simulink model "gm_Sementation_8K"  (R2019a)
settings: Solver=FixedStepDiscrete  StartTime=0.0  StopTime=Ts_240p*20  RelTol=1e-3
InitFcn:
  | Ts = 1e-3;
  | Ts_240p = 402*324*Ts;
  | Ts_480p = 525*800*Ts;
undefined symbols (not defined in the file or in its folder): gray, Rec, SDTV
libraries: hdlsllib x14, visionhdlio x2, visionhdlconversions x2, dspvision x1
settings Model: ModifiedByFormat=The MathWorks Inc.  Creator=The MathWorks, Inc.  LastModifiedBy=The MathWorks Inc.
settings DataIOCC: LimitDataPoints=on  SaveFormat=Array  SaveOutput=off  SaveTime=off  ReturnWorkspaceOutputs=off
settings OptimizationCC: BlockReduction=off  ConditionallyExecuteInputs=off  DefaultParameterBehavior=Inlined  LifeSpan=inf
settings DebuggingCC: AlgebraicLoopMsg=error  SolverPrmCheckMsg=warning  InheritedTsInSrcMsg=none  SingleTaskRateTransMsg=error  ParameterPrecisionLossMsg=none  AllowSymbolicDim=off  SFUnexpectedBacktrackingDiag=warning  SFNoUnconditionalDefaultTransitionDiag=warning  SFExecutionAtInitializationDiag=none  IntegerSaturationMsg=none  ArithmeticOperatorsInVariantConditions=warning
settings HardwareCC: ProdBitPerPointer=32  ProdBitPerSizeT=32  ProdBitPerPtrDiffT=32  ProdLargestAtomicFloat=None  ProdIntDivRoundTo=Undefined  ProdEndianess=Unspecified  ProdWordSize=32  ProdHWDeviceType=ASIC/FPGA->ASIC/FPGA  ProdEqTarget=off
settings ModelReferenceCC: PropagateSignalLabelsOutOfModel=off
settings SFSimCC: SimUseLocalCustomCode=off
settings RTWCC: RTWUseLocalCustomCode=off
settings CodeAppCC: StateflowObjectComments=on
settings GRTTargetCC: TargetLangStandard=C89/C90 (ANSI)  GeneratePreprocessorConditionals=Disable all
settings ConfigComp: CovMetricSettings=dw  CovHtmlReporting=on  CovSaveCumulativeToWorkspaceVar=on  CovSaveSingleToWorkspaceVar=on  CovShowResultsExplorer=off  CovExternalEMLEnable=off  CovSFcnEnable=off

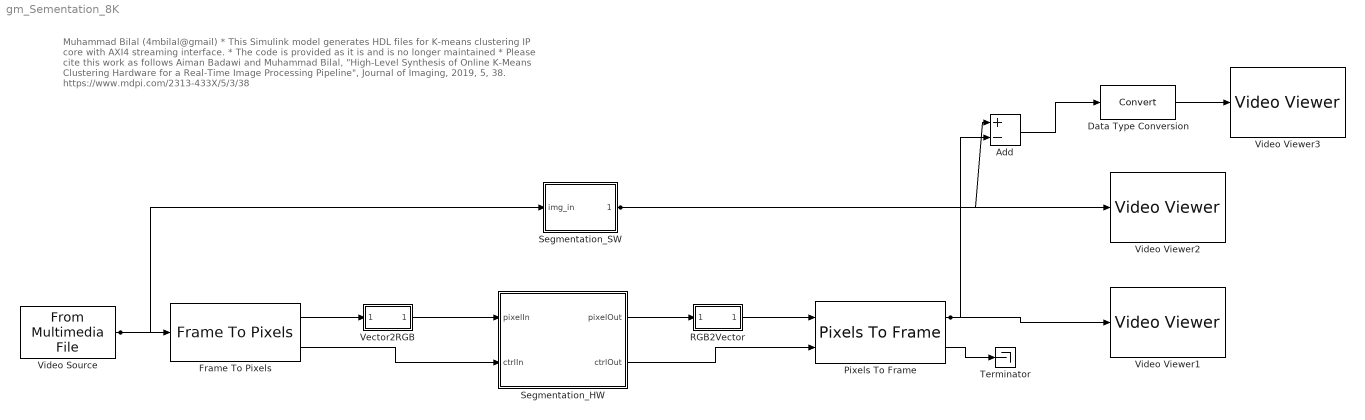
== system gm_Sementation_8K ==
  note: Muhammad Bilal (4mbilal@gmail)
      |
      | * This Simulink model generates HDL files for K-means clustering IP core with AXI4 streaming interface.
      |
      | * The code is provided as it is and is no longer maintained
      |
      | * Please cite this work as follows
      | Aiman Badawi and Muhammad Bilal, "High-Level Synthesis of Online K-Means Clustering Hardware for a Real-Time Image Processing Pipeline", Journal of Imaging, 2019, 5, 38.
      | https://www.mdpi.com/2313-433X/5/3/38
  Add : Sum  Inputs=+-
  Data Type Conversion : DataTypeConversion
  Frame To Pixels : visionhdlio/Frame To Pixels  NumComponents=3  VideoFormat=240p  ActivePixelsPerLine=32  ActiveVideoLines=18  TotalPixelsPerLine=42  TotalVideoLines=28  StartingActiveLine=6  FrontPorch=5  SampleTime=0
      settings: SourceProductName=Vision HDL Toolbox  SourceProductBaseCode=VT
  Pixels To Frame : visionhdlio/Pixels To Frame  NumComponents=3  VideoFormat=240p  ActivePixelsPerLine=32  ActiveVideoLines=18  TotalPixelsPerLine=42  TotalVideoLines=28
      settings: SourceProductName=Vision HDL Toolbox  SourceProductBaseCode=VT
  RGB2Vector : Subsystem
  Segmentation_HW : Subsystem  TreatAsAtomicUnit=on
  Segmentation_SW : MATLAB Function  TreatAsAtomicUnit=on
  Terminator : Terminator
  Vector2RGB : Subsystem
  Video Source : dspvision/From Multimedia File  inputFilename=E:\RnD\Current_Projects\Musawwir\Frameworks\HW\Musawwir_HW_Zedboard\Custom_IP_Cores\Matlab\Segmentation\images\mountain.jpg  readRange=[1 Inf]  loop=on  numPlays=inf  outputStreams=Video only  videoDataType=uint8  audioDataType=int16  inheritSampleTime=off  userDefinedSampleTime=Ts_240p  noAudioOutput=off  isIntensityVideo=off  fourcc=RGB  colorVideoFormat=One multidimensional signal  outputEOF=off  dataOrg=Column-major  audioFrameSize=1024  computeAudioFrameSize=off  outSamplingMode=Sample based
      settings: SourceProductName=Computer Vision Toolbox  SourceProductBaseCode=VP
  Video Viewer1 : VideoViewer  colormapValue=gray(256)  FigPos=[54.6 658.8 498.4 402.4]
  Video Viewer2 : VideoViewer  colormapValue=gray(256)  FigPos=[554.6 659.6 498.4 402.4]
  Video Viewer3 : VideoViewer  colormapValue=gray(256)  FigPos=[1020.2 514 498.4 402.4]
  wires:
  Data Type Conversion/1 -> Video Viewer3/1
  Add/1 -> Data Type Conversion/1
  Segmentation_SW/1(img_out) -> Video Viewer2/1, Add/1
  Segmentation_HW/2(ctrlOut) -> Pixels To Frame/2
  RGB2Vector/1(RGBVector) -> Pixels To Frame/1
  Frame To Pixels/1 -> Vector2RGB/1(RGBVector)
  Frame To Pixels/2 -> Segmentation_HW/2(ctrlIn)
  Video Source/1 -> Frame To Pixels/1, Segmentation_SW/1(img_in)
  Segmentation_HW/1(pixelOut) -> RGB2Vector/1(RGB)
  Vector2RGB/1(RGB) -> Segmentation_HW/1(pixelIn)
  Pixels To Frame/1 -> Video Viewer1/1, Add/2
  Pixels To Frame/2 -> Terminator/1

== system gm_Sementation_8K/RGB2Vector ==
  note: RGB represented in
      | 32'hFFRRGGBB
  RGB : Inport
  Bit Slice : hdlsllib/Logic and Bit Operations/Bit Slice  lidx=23  ridx=16
  Bit Slice1 : hdlsllib/Logic and Bit Operations/Bit Slice  lidx=15  ridx=8
  Bit Slice2 : hdlsllib/Logic and Bit Operations/Bit Slice  lidx=7  ridx=0
  Mux : Mux  Inputs=3
  Signal Specification : SignalSpecification
  Transpose : Math  Operator=transpose  SaturateOnIntegerOverflow=on
  RGBVector : Outport
  wires:
  Signal Specification/1 -> RGBVector/1
  Transpose/1 -> Signal Specification/1
  RGB/1 -> Bit Slice/1, Bit Slice1/1, Bit Slice2/1
  Bit Slice1/1 -> Mux/2
  Bit Slice2/1 -> Mux/3
  Bit Slice/1 -> Mux/1
  Mux/1 -> Transpose/1

== system gm_Sementation_8K/Segmentation_HW ==
  pixelIn : Inport  OutDataTypeStr=uint32  PortDimensions=1  SampleTime=0.001
  ctrlIn : Inport  Port=2  SampleTime=0.001
  Bit Concat : hdlsllib/Logic and Bit Operations/Bit Concat  numInputs=4
      settings: SourceProductName=HDL Coder  SourceProductBaseCode=HD
  Demux : Demux  Outputs=3
  FF : Constant  Value=255  OutDataTypeStr=uint8  SampleTime=Ts
  K-Means : Subsystem
  RGB2Vector : Subsystem
  pixelOut : Outport
  ctrlOut : Outport  Port=2
  wires:
  pixelIn/1 -> RGB2Vector/1(RGB)
  ctrlIn/1 -> K-Means/2(ctrlIn)
  Bit Concat/1 -> pixelOut/1
  Demux/1 -> Bit Concat/2
  Demux/2 -> Bit Concat/3
  Demux/3 -> Bit Concat/4
  FF/1 -> Bit Concat/1
  K-Means/1(pixelOut) -> Demux/1
  K-Means/2(ctrlOut) -> ctrlOut/1
  RGB2Vector/1(RGBVector) -> K-Means/1(pixelIn)

== system gm_Sementation_8K/Vector2RGB ==
  note: Encode RGB into 32 bit representation
      | 32'hFFRRGGBB
  RGBVector : Inport
  Bit Concat : hdlsllib/Logic and Bit Operations/Bit Concat  numInputs=4
      settings: SourceProductName=HDL Coder  SourceProductBaseCode=HD
  Demux : Demux  Outputs=3
  FF : Constant  Value=255  OutDataTypeStr=uint8  SampleTime=Ts
  RGB : Outport
  wires:
  Demux/3 -> Bit Concat/4
  Demux/2 -> Bit Concat/3
  Demux/1 -> Bit Concat/2
  FF/1 -> Bit Concat/1
  RGBVector/1 -> Demux/1
  Bit Concat/1 -> RGB/1

== system gm_Sementation_8K/Segmentation_HW/K-Means ==
  pixelIn : Inport  OutDataTypeStr=uint8  PortDimensions=[3]  SampleTime=0.001
  ctrlIn : Inport  Port=2  SampleTime=0.001
  Clustering : Subsystem
  Color Space Converter : visionhdlconversions/Color Space Converter  Conversion=RGB to YCbCr  ConversionStandard=Rec. 601 (SDTV)  ScanningStandard=1250/50/2:1  SimulateUsing=Code generation
      settings: SourceProductName=Vision HDL Toolbox  SourceProductBaseCode=VT
  Color Space Converter1 : visionhdlconversions/Color Space Converter  Conversion=YCbCr to RGB  ConversionStandard=Rec. 601 (SDTV)  ScanningStandard=1250/50/2:1  SimulateUsing=Code generation
      settings: SourceProductName=Vision HDL Toolbox  SourceProductBaseCode=VT
  Comparisons : Subsystem
  Data Type Conversion1 : DataTypeConversion  OutDataTypeStr=uint8  RndMeth=Nearest  SampleTime=0.001
  Data Type Conversion2 : DataTypeConversion  OutDataTypeStr=fixdt(1, 18, 8)  RndMeth=Nearest  SampleTime=0.001
  pixelOut : Outport
  ctrlOut : Outport  Port=2
  wires:
  pixelIn/1 -> Color Space Converter/1
  ctrlIn/1 -> Color Space Converter/2
  Clustering/1(K_out) -> Comparisons/2(Ks)
  Color Space Converter/1 -> Data Type Conversion2/1
  Color Space Converter/2 -> Clustering/3(Ctrl), Color Space Converter1/2
  Color Space Converter1/1 -> pixelOut/1
  Color Space Converter1/2 -> ctrlOut/1
  Comparisons/1(K_out) -> Data Type Conversion1/1
  Comparisons/2(Address) -> Clustering/1(K_addr)
  Data Type Conversion1/1 -> Color Space Converter1/1
  Data Type Conversion2/1 -> Clustering/2(RGB_pixel), Comparisons/1(RGB_pixel)

== system gm_Sementation_8K/Segmentation_HW/RGB2Vector ==
  RGB : Inport  OutDataTypeStr=uint32  PortDimensions=1  SampleTime=0.001
  Bit Slice : hdlsllib/Logic and Bit Operations/Bit Slice  lidx=23  ridx=16
  Bit Slice1 : hdlsllib/Logic and Bit Operations/Bit Slice  lidx=15  ridx=8
  Bit Slice2 : hdlsllib/Logic and Bit Operations/Bit Slice  lidx=7  ridx=0
  Mux : Mux  Inputs=3
  RGBVector : Outport
  wires:
  RGB/1 -> Bit Slice2/1, Bit Slice1/1, Bit Slice/1
  Bit Slice/1 -> Mux/1
  Bit Slice1/1 -> Mux/2
  Bit Slice2/1 -> Mux/3
  Mux/1 -> RGBVector/1

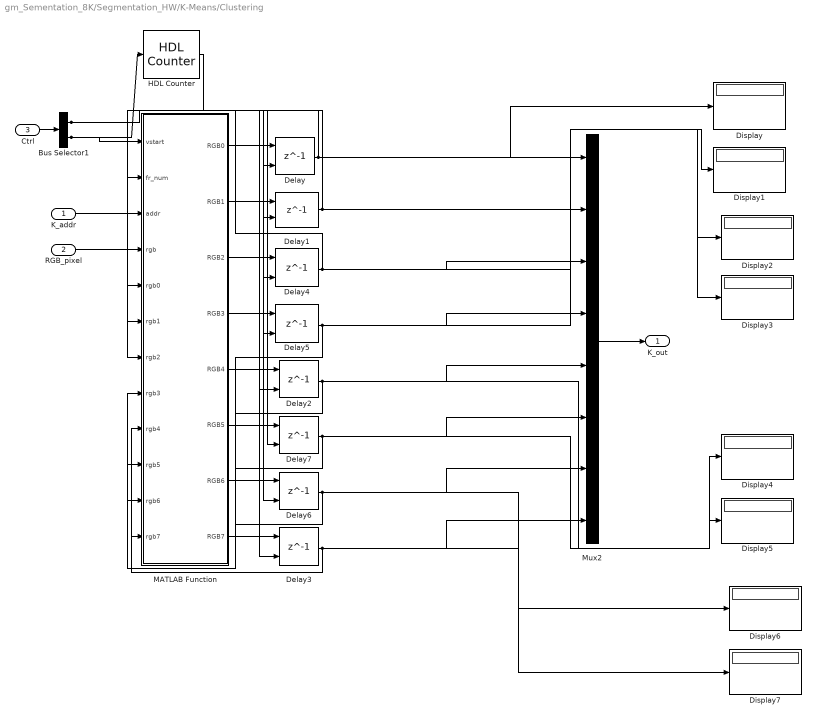
== system gm_Sementation_8K/Segmentation_HW/K-Means/Clustering ==
  K_addr : Inport  OutDataTypeStr=fixdt(0, 3, 0)  PortDimensions=1  SampleTime=0.001
  RGB_pixel : Inport  Port=2  OutDataTypeStr=fixdt(1, 18, 8)  PortDimensions=[1 3]  SampleTime=0.001
  Ctrl : Inport  Port=3  SampleTime=0.001
  Bus Selector1 : BusSelector  OutputSignals=valid,vStart
  Delay{,1..7} (8 alike) : Delay  DelayLength=1  InitialCondition=0  ShowEnablePort=on
      settings: InputPortMap=u0,e6
  Display{,1..7} (8 alike) : Display
  HDL Counter : hdlsllib/Sources/HDL Counter  CountType=Free running  CountInit=0  CountStep=1  CountMax=4  CountFromType=Initial value  CountFrom=0  CountResetPort=off  CountLoadPort=off  CountEnbPort=on  CountDirPort=off  CountDataType=Unsigned  CountWordLen=12  CountFracLen=0  CountSampTime=1
      settings: SourceProductBaseCode=HD
  MATLAB Function : Subsystem
  Mux2 : Mux  Inputs=8
  K_out : Outport
  wires:
  K_addr/1 -> MATLAB Function/3(addr)
  RGB_pixel/1 -> MATLAB Function/4(rgb)
  Ctrl/1 -> Bus Selector1/1
  Bus Selector1/1 -> Delay7/2, Delay6/2, Delay5/2, Delay4/2, Delay3/2, Delay2/2, Delay1/2, Delay/2
  Bus Selector1/2 -> HDL Counter/1, MATLAB Function/1(vstart)
  Delay/1 -> Mux2/1, Display/1, MATLAB Function/5(rgb0)
  Delay1/1 -> Mux2/2, Display1/1, MATLAB Function/6(rgb1)
  Delay2/1 -> Mux2/5, Display4/1, MATLAB Function/9(rgb4)
  Delay3/1 -> Mux2/8, Display7/1, MATLAB Function/12(rgb7)
  Delay4/1 -> Mux2/3, Display2/1, MATLAB Function/7(rgb2)
  Delay5/1 -> Mux2/4, Display3/1, MATLAB Function/8(rgb3)
  Delay6/1 -> Mux2/7, Display6/1, MATLAB Function/11(rgb6)
  Delay7/1 -> Mux2/6, Display5/1, MATLAB Function/10(rgb5)
  HDL Counter/1 -> MATLAB Function/2(fr_num)
  MATLAB Function/1(RGB0) -> Delay/1
  MATLAB Function/2(RGB1) -> Delay1/1
  MATLAB Function/3(RGB2) -> Delay4/1
  MATLAB Function/4(RGB3) -> Delay5/1
  MATLAB Function/5(RGB4) -> Delay2/1
  MATLAB Function/6(RGB5) -> Delay7/1
  MATLAB Function/7(RGB6) -> Delay6/1
  MATLAB Function/8(RGB7) -> Delay3/1
  Mux2/1 -> K_out/1

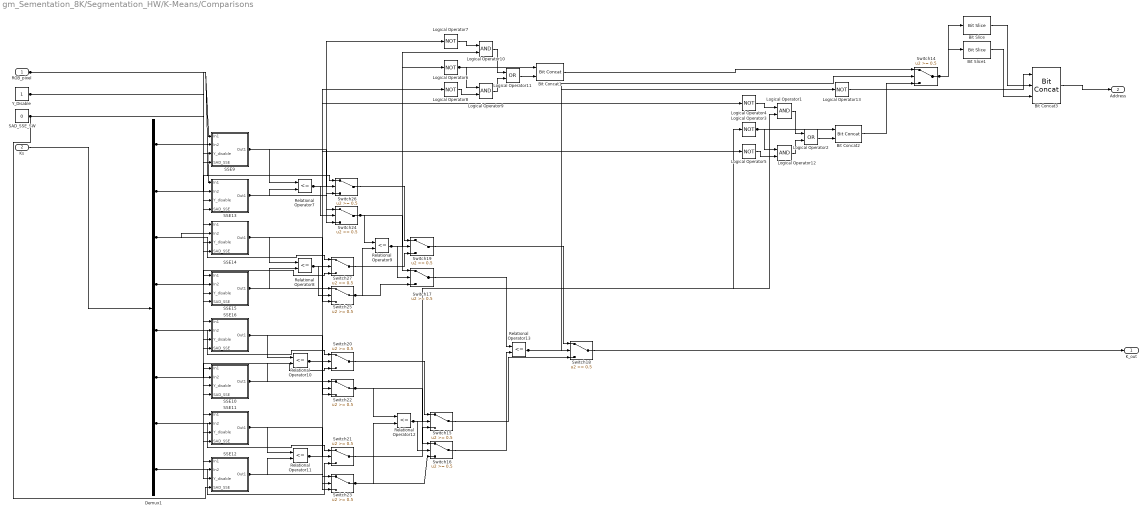
== system gm_Sementation_8K/Segmentation_HW/K-Means/Comparisons ==
  RGB_pixel : Inport  OutDataTypeStr=fixdt(1, 18, 8)  PortDimensions=[1 3]  SampleTime=0.001
  Ks : Inport  Port=2  OutDataTypeStr=fixdt(1, 18, 8)  PortDimensions=[1 24]  SampleTime=0.001
  Bit Concat1 : hdlsllib/Logic and Bit Operations/Bit Concat  numInputs=2
      settings: SourceProductName=HDL Coder  SourceProductBaseCode=HD
  Bit Concat2 : hdlsllib/Logic and Bit Operations/Bit Concat  numInputs=2
      settings: SourceProductName=HDL Coder  SourceProductBaseCode=HD
  Bit Concat3 : hdlsllib/Logic and Bit Operations/Bit Concat  numInputs=3
      settings: SourceProductName=HDL Coder  SourceProductBaseCode=HD
  Bit Slice : hdlsllib/Logic and Bit Operations/Bit Slice  lidx=1  ridx=1
  Bit Slice1 : hdlsllib/Logic and Bit Operations/Bit Slice  lidx=0  ridx=0
  Demux1 : Demux  Outputs=8
  Logical Operator{1,9..10,12} (4 alike) : Logic  AllPortsSameDT=off  OutDataTypeStr=boolean
  Logical Operator11 : Logic  Operator=OR  AllPortsSameDT=off  OutDataTypeStr=boolean
  Logical Operator{3..8,13} (7 alike) : Logic  Operator=NOT  AllPortsSameDT=off  OutDataTypeStr=boolean
  Logical Operator2 : Logic  Operator=OR  AllPortsSameDT=off  OutDataTypeStr=boolean
  Relational Operator{7..13} (7 alike) : RelationalOperator  Operator=<=  OutDataTypeStr=boolean  RndMeth=Nearest
  SAD_SSE_SW : Constant  Value=0  OutDataTypeStr=fixdt(1,18,8)
  SSE10 : Subsystem
  SSE11 : Subsystem
  SSE12 : Subsystem
  SSE13 : Subsystem
  SSE14 : Subsystem
  SSE15 : Subsystem
  SSE16 : Subsystem
  SSE9 : Subsystem
  Switch{14..27} (14 alike) : Switch  Threshold=0.5
  Y_Disable : Constant  OutDataTypeStr=fixdt(1,18,8)
  K_out : Outport
  Address : Outport  Port=2
  wires:
  RGB_pixel/1 -> SSE13/1(In1), SSE14/1(In1), SSE11/1(In1), SSE12/1(In1), SSE10/1(In1), SSE16/1(In1), SSE15/1(In1), SSE9/1(In1)
  Ks/1 -> Demux1/1
  Bit Concat1/1 -> Switch14/1
  Bit Concat2/1 -> Switch14/3
  Bit Concat3/1 -> Address/1
  Bit Slice/1 -> Bit Concat3/2
  Bit Slice1/1 -> Bit Concat3/3
  Demux1/1 -> Switch26/1, SSE9/2(In2)
  Demux1/2 -> Switch26/3, SSE13/2(In2)
  Demux1/3 -> Switch27/1, SSE14/2(In2)
  Demux1/4 -> Switch27/3, SSE15/2(In2)
  Demux1/5 -> Switch20/1, SSE16/2(In2)
  Demux1/6 -> Switch20/3, SSE10/2(In2)
  Demux1/7 -> Switch21/1, SSE11/2(In2)
  Demux1/8 -> Switch21/3, SSE12/2(In2)
  Logical Operator1/1 -> Logical Operator2/1
  Logical Operator10/1 -> Logical Operator11/1
  Logical Operator11/1 -> Bit Concat1/2
  Logical Operator12/1 -> Logical Operator2/2
  Logical Operator13/1 -> Bit Concat3/1
  Logical Operator2/1 -> Bit Concat2/2
  Logical Operator3/1 -> Logical Operator12/1, Bit Concat2/1
  Logical Operator4/1 -> Logical Operator1/1
  Logical Operator5/1 -> Logical Operator12/2
  Logical Operator6/1 -> Logical Operator9/1, Bit Concat1/1
  Logical Operator7/1 -> Logical Operator10/1
  Logical Operator8/1 -> Logical Operator9/2
  Logical Operator9/1 -> Logical Operator11/2
  Relational Operator10/1 -> Switch22/2, Switch20/2, Logical Operator4/1
  Relational Operator11/1 -> Switch23/2, Switch21/2, Logical Operator5/1
  Relational Operator12/1 -> Switch16/2, Switch15/2, Logical Operator3/1, Logical Operator1/2
  Relational Operator13/1 -> Switch18/2, Switch14/2, Logical Operator13/1
  Relational Operator7/1 -> Switch26/2, Switch24/2, Logical Operator7/1
  Relational Operator8/1 -> Switch27/2, Switch25/2, Logical Operator8/1
  Relational Operator9/1 -> Switch19/2, Switch17/2, Logical Operator6/1, Logical Operator10/2
  SAD_SSE_SW/1 -> SSE12/4(SAD_SSE), SSE11/4(SAD_SSE), SSE10/4(SAD_SSE), SSE16/4(SAD_SSE), SSE15/4(SAD_SSE), SSE14/4(SAD_SSE), SSE13/4(SAD_SSE), SSE9/4(SAD_SSE)
  SSE10/1(Out1) -> Switch22/3, Relational Operator10/2
  SSE11/1(Out1) -> Switch23/1, Relational Operator11/1
  SSE12/1(Out1) -> Switch23/3, Relational Operator11/2
  SSE13/1(Out1) -> Switch24/3, Relational Operator7/2
  SSE14/1(Out1) -> Switch25/1, Relational Operator8/1
  SSE15/1(Out1) -> Switch25/3, Relational Operator8/2
  SSE16/1(Out1) -> Switch22/1, Relational Operator10/1
  SSE9/1(Out1) -> Switch24/1, Relational Operator7/1
  Switch14/1 -> Bit Slice1/1, Bit Slice/1
  Switch15/1 -> Switch18/3
  Switch16/1 -> Relational Operator13/2
  Switch17/1 -> Relational Operator13/1
  Switch18/1 -> K_out/1
  Switch19/1 -> Switch18/1
  Switch20/1 -> Switch15/1
  Switch21/1 -> Switch15/3
  Switch22/1 -> Switch16/1, Relational Operator12/1
  Switch23/1 -> Switch16/3, Relational Operator12/2
  Switch24/1 -> Switch17/1, Relational Operator9/1
  Switch25/1 -> Switch17/3, Relational Operator9/2
  Switch26/1 -> Switch19/1
  Switch27/1 -> Switch19/3
  Y_Disable/1 -> SSE9/3(Y_disable), SSE13/3(Y_disable), SSE16/3(Y_disable), SSE11/3(Y_disable), SSE12/3(Y_disable), SSE10/3(Y_disable), SSE15/3(Y_disable), SSE14/3(Y_disable)

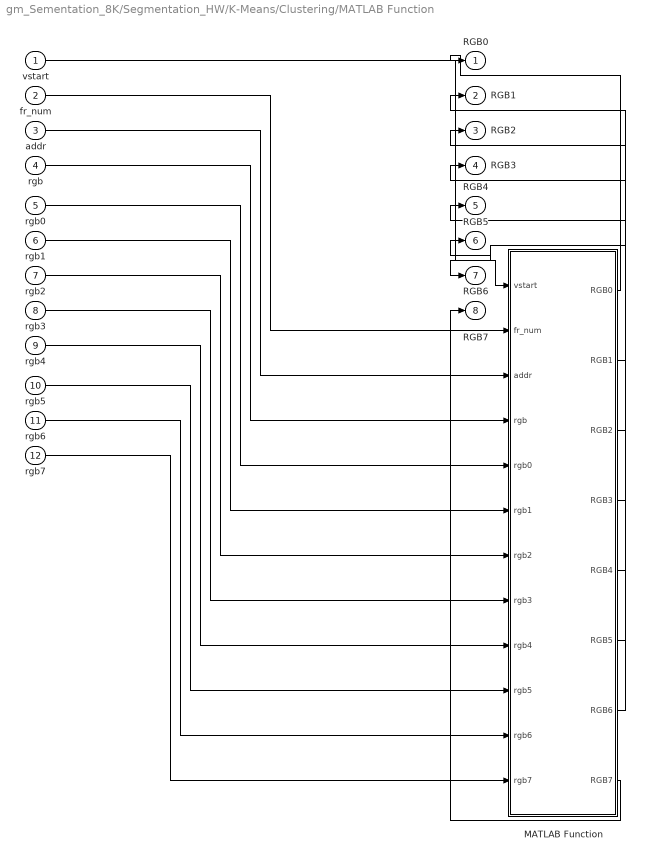
== system gm_Sementation_8K/Segmentation_HW/K-Means/Clustering/MATLAB Function ==
  vstart : Inport  OutDataTypeStr=boolean  PortDimensions=1  SampleTime=0.001
  fr_num : Inport  Port=2  OutDataTypeStr=fixdt(0, 12, 0)  PortDimensions=1  SampleTime=0.001
  addr : Inport  Port=3  OutDataTypeStr=fixdt(0, 3, 0)  PortDimensions=1  SampleTime=0.001
  rgb : Inport  Port=4  OutDataTypeStr=fixdt(1, 18, 8)  PortDimensions=[1 3]  SampleTime=0.001
  rgb0 : Inport  Port=5  OutDataTypeStr=fixdt(1, 18, 8)  PortDimensions=[1 3]  SampleTime=0.001
  rgb1 : Inport  Port=6  OutDataTypeStr=fixdt(1, 18, 8)  PortDimensions=[1 3]  SampleTime=0.001
  rgb2 : Inport  Port=7  OutDataTypeStr=fixdt(1, 18, 8)  PortDimensions=[1 3]  SampleTime=0.001
  rgb3 : Inport  Port=8  OutDataTypeStr=fixdt(1, 18, 8)  PortDimensions=[1 3]  SampleTime=0.001
  rgb4 : Inport  Port=9  OutDataTypeStr=fixdt(1, 18, 8)  PortDimensions=[1 3]  SampleTime=0.001
  rgb5 : Inport  Port=10  OutDataTypeStr=fixdt(1, 18, 8)  PortDimensions=[1 3]  SampleTime=0.001
  rgb6 : Inport  Port=11  OutDataTypeStr=fixdt(1, 18, 8)  PortDimensions=[1 3]  SampleTime=0.001
  rgb7 : Inport  Port=12  OutDataTypeStr=fixdt(1, 18, 8)  PortDimensions=[1 3]  SampleTime=0.001
  MATLAB Function : MATLAB Function  TreatAsAtomicUnit=on
  RGB0 : Outport
  RGB1 : Outport  Port=2
  RGB2 : Outport  Port=3
  RGB3 : Outport  Port=4
  RGB4 : Outport  Port=5
  RGB5 : Outport  Port=6
  RGB6 : Outport  Port=7
  RGB7 : Outport  Port=8
  wires:
  vstart/1 -> MATLAB Function/1(vstart)
  fr_num/1 -> MATLAB Function/2(fr_num)
  addr/1 -> MATLAB Function/3(addr)
  rgb/1 -> MATLAB Function/4(rgb)
  rgb0/1 -> MATLAB Function/5(rgb0)
  rgb1/1 -> MATLAB Function/6(rgb1)
  rgb2/1 -> MATLAB Function/7(rgb2)
  rgb3/1 -> MATLAB Function/8(rgb3)
  rgb4/1 -> MATLAB Function/9(rgb4)
  rgb5/1 -> MATLAB Function/10(rgb5)
  rgb6/1 -> MATLAB Function/11(rgb6)
  rgb7/1 -> MATLAB Function/12(rgb7)
  MATLAB Function/1(RGB0) -> RGB0/1
  MATLAB Function/2(RGB1) -> RGB1/1
  MATLAB Function/3(RGB2) -> RGB2/1
  MATLAB Function/4(RGB3) -> RGB3/1
  MATLAB Function/5(RGB4) -> RGB4/1
  MATLAB Function/6(RGB5) -> RGB5/1
  MATLAB Function/7(RGB6) -> RGB6/1
  MATLAB Function/8(RGB7) -> RGB7/1

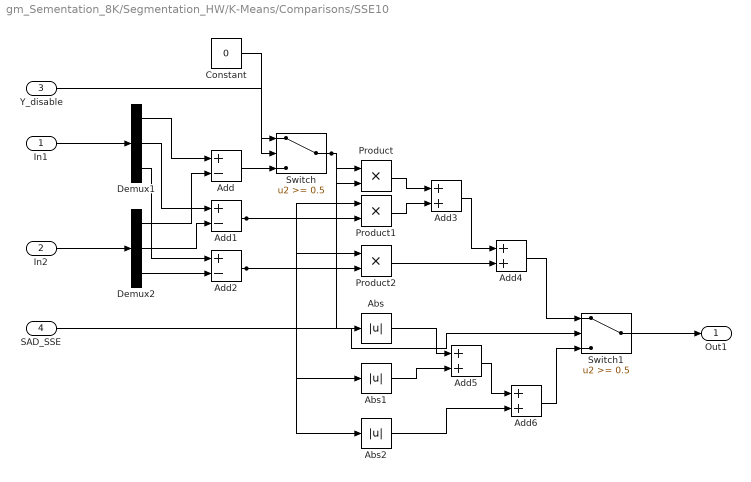
== system gm_Sementation_8K/Segmentation_HW/K-Means/Comparisons/SSE10 ==
  In1 : Inport  OutDataTypeStr=fixdt(1, 18, 8)  PortDimensions=[1 3]  SampleTime=0.001
  In2 : Inport  Port=2  OutDataTypeStr=fixdt(1, 18, 8)  PortDimensions=[1 3]  SampleTime=0.001
  Y_disable : Inport  Port=3  OutDataTypeStr=fixdt(1, 18, 8)  PortDimensions=1
  SAD_SSE : Inport  Port=4  OutDataTypeStr=fixdt(1, 18, 8)  PortDimensions=1
  Abs : Abs
  Abs1 : Abs
  Abs2 : Abs
  Add : Sum  Inputs=+-  OutDataTypeStr=Inherit: Inherit via back propagation
  Add1 : Sum  Inputs=+-  OutDataTypeStr=Inherit: Inherit via back propagation
  Add2 : Sum  Inputs=+-  OutDataTypeStr=Inherit: Inherit via back propagation
  Add{3..6} (4 alike) : Sum
  Constant : Constant  Value=0  OutDataTypeStr=fixdt(1,18,8)
  Demux1 : Demux  Outputs=3
  Demux2 : Demux  Outputs=3
  Product : Product
  Product1 : Product
  Product2 : Product
  Switch : Switch  Threshold=0.5
  Switch1 : Switch  Threshold=0.5
  Out1 : Outport
  wires:
  In1/1 -> Demux1/1
  In2/1 -> Demux2/1
  Y_disable/1 -> Switch/2
  SAD_SSE/1 -> Switch1/2
  Abs/1 -> Add5/1
  Abs1/1 -> Add5/2
  Abs2/1 -> Add6/2
  Add/1 -> Switch/3
  Add1/1 -> Product1/2, Product1/1, Abs1/1
  Add2/1 -> Product2/2, Product2/1, Abs2/1
  Add3/1 -> Add4/1
  Add4/1 -> Switch1/1
  Add5/1 -> Add6/1
  Add6/1 -> Switch1/3
  Constant/1 -> Switch/1
  Demux1/1 -> Add/1
  Demux1/2 -> Add1/1
  Demux1/3 -> Add2/1
  Demux2/1 -> Add/2
  Demux2/2 -> Add1/2
  Demux2/3 -> Add2/2
  Product/1 -> Add3/1
  Product1/1 -> Add3/2
  Product2/1 -> Add4/2
  Switch/1 -> Product/2, Product/1, Abs/1
  Switch1/1 -> Out1/1

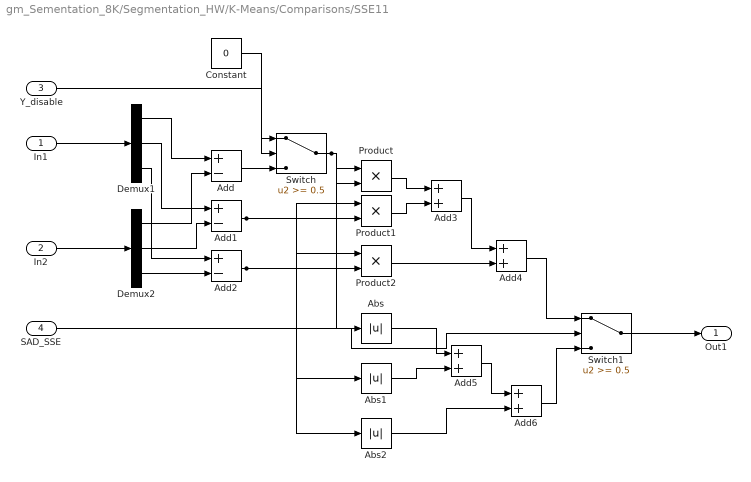
== system gm_Sementation_8K/Segmentation_HW/K-Means/Comparisons/SSE11 ==
  In1 : Inport  OutDataTypeStr=fixdt(1, 18, 8)  PortDimensions=[1 3]  SampleTime=0.001
  In2 : Inport  Port=2  OutDataTypeStr=fixdt(1, 18, 8)  PortDimensions=[1 3]  SampleTime=0.001
  Y_disable : Inport  Port=3  OutDataTypeStr=fixdt(1, 18, 8)  PortDimensions=1
  SAD_SSE : Inport  Port=4  OutDataTypeStr=fixdt(1, 18, 8)  PortDimensions=1
  Abs : Abs
  Abs1 : Abs
  Abs2 : Abs
  Add : Sum  Inputs=+-  OutDataTypeStr=Inherit: Inherit via back propagation
  Add1 : Sum  Inputs=+-  OutDataTypeStr=Inherit: Inherit via back propagation
  Add2 : Sum  Inputs=+-  OutDataTypeStr=Inherit: Inherit via back propagation
  Add{3..6} (4 alike) : Sum
  Constant : Constant  Value=0  OutDataTypeStr=fixdt(1,18,8)
  Demux1 : Demux  Outputs=3
  Demux2 : Demux  Outputs=3
  Product : Product
  Product1 : Product
  Product2 : Product
  Switch : Switch  Threshold=0.5
  Switch1 : Switch  Threshold=0.5
  Out1 : Outport
  wires:
  In1/1 -> Demux1/1
  In2/1 -> Demux2/1
  Y_disable/1 -> Switch/2
  SAD_SSE/1 -> Switch1/2
  Abs/1 -> Add5/1
  Abs1/1 -> Add5/2
  Abs2/1 -> Add6/2
  Add/1 -> Switch/3
  Add1/1 -> Product1/2, Product1/1, Abs1/1
  Add2/1 -> Product2/2, Product2/1, Abs2/1
  Add3/1 -> Add4/1
  Add4/1 -> Switch1/1
  Add5/1 -> Add6/1
  Add6/1 -> Switch1/3
  Constant/1 -> Switch/1
  Demux1/1 -> Add/1
  Demux1/2 -> Add1/1
  Demux1/3 -> Add2/1
  Demux2/1 -> Add/2
  Demux2/2 -> Add1/2
  Demux2/3 -> Add2/2
  Product/1 -> Add3/1
  Product1/1 -> Add3/2
  Product2/1 -> Add4/2
  Switch/1 -> Product/2, Product/1, Abs/1
  Switch1/1 -> Out1/1

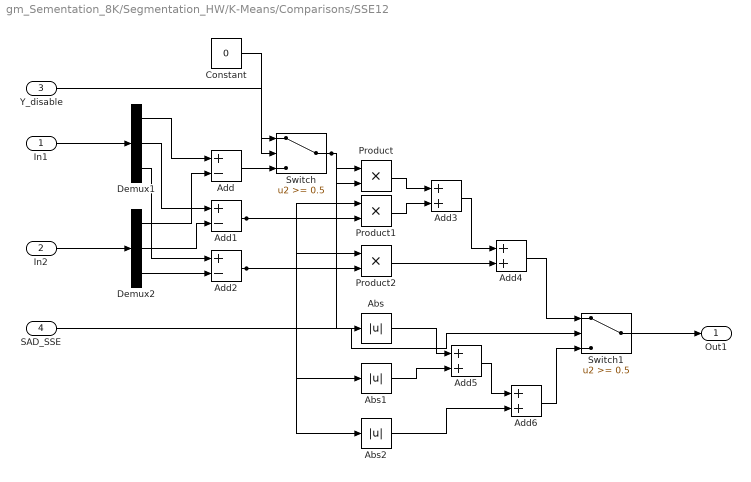
== system gm_Sementation_8K/Segmentation_HW/K-Means/Comparisons/SSE12 ==
  In1 : Inport  OutDataTypeStr=fixdt(1, 18, 8)  PortDimensions=[1 3]  SampleTime=0.001
  In2 : Inport  Port=2  OutDataTypeStr=fixdt(1, 18, 8)  PortDimensions=[1 3]  SampleTime=0.001
  Y_disable : Inport  Port=3  OutDataTypeStr=fixdt(1, 18, 8)  PortDimensions=1
  SAD_SSE : Inport  Port=4  OutDataTypeStr=fixdt(1, 18, 8)  PortDimensions=1
  Abs : Abs
  Abs1 : Abs
  Abs2 : Abs
  Add : Sum  Inputs=+-  OutDataTypeStr=Inherit: Inherit via back propagation
  Add1 : Sum  Inputs=+-  OutDataTypeStr=Inherit: Inherit via back propagation
  Add2 : Sum  Inputs=+-  OutDataTypeStr=Inherit: Inherit via back propagation
  Add{3..6} (4 alike) : Sum
  Constant : Constant  Value=0  OutDataTypeStr=fixdt(1,18,8)
  Demux1 : Demux  Outputs=3
  Demux2 : Demux  Outputs=3
  Product : Product
  Product1 : Product
  Product2 : Product
  Switch : Switch  Threshold=0.5
  Switch1 : Switch  Threshold=0.5
  Out1 : Outport
  wires:
  In1/1 -> Demux1/1
  In2/1 -> Demux2/1
  Y_disable/1 -> Switch/2
  SAD_SSE/1 -> Switch1/2
  Abs/1 -> Add5/1
  Abs1/1 -> Add5/2
  Abs2/1 -> Add6/2
  Add/1 -> Switch/3
  Add1/1 -> Product1/2, Product1/1, Abs1/1
  Add2/1 -> Product2/2, Product2/1, Abs2/1
  Add3/1 -> Add4/1
  Add4/1 -> Switch1/1
  Add5/1 -> Add6/1
  Add6/1 -> Switch1/3
  Constant/1 -> Switch/1
  Demux1/1 -> Add/1
  Demux1/2 -> Add1/1
  Demux1/3 -> Add2/1
  Demux2/1 -> Add/2
  Demux2/2 -> Add1/2
  Demux2/3 -> Add2/2
  Product/1 -> Add3/1
  Product1/1 -> Add3/2
  Product2/1 -> Add4/2
  Switch/1 -> Product/2, Product/1, Abs/1
  Switch1/1 -> Out1/1

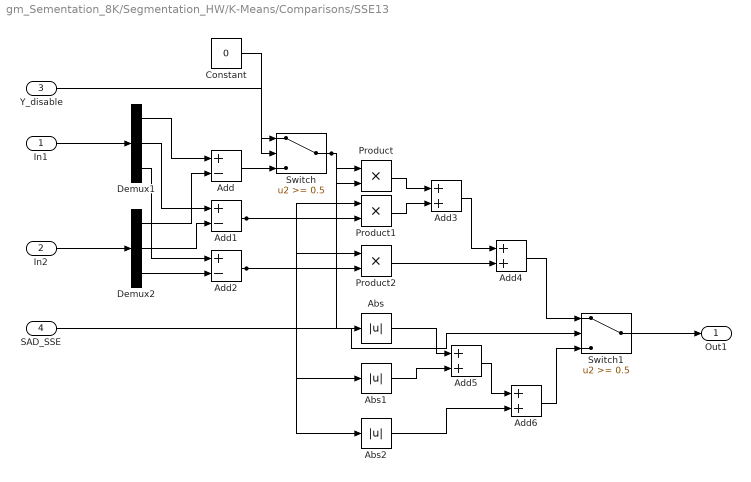
== system gm_Sementation_8K/Segmentation_HW/K-Means/Comparisons/SSE13 ==
  In1 : Inport  OutDataTypeStr=fixdt(1, 18, 8)  PortDimensions=[1 3]  SampleTime=0.001
  In2 : Inport  Port=2  OutDataTypeStr=fixdt(1, 18, 8)  PortDimensions=[1 3]  SampleTime=0.001
  Y_disable : Inport  Port=3  OutDataTypeStr=fixdt(1, 18, 8)  PortDimensions=1
  SAD_SSE : Inport  Port=4  OutDataTypeStr=fixdt(1, 18, 8)  PortDimensions=1
  Abs : Abs
  Abs1 : Abs
  Abs2 : Abs
  Add : Sum  Inputs=+-  OutDataTypeStr=Inherit: Inherit via back propagation
  Add1 : Sum  Inputs=+-  OutDataTypeStr=Inherit: Inherit via back propagation
  Add2 : Sum  Inputs=+-  OutDataTypeStr=Inherit: Inherit via back propagation
  Add{3..6} (4 alike) : Sum
  Constant : Constant  Value=0  OutDataTypeStr=fixdt(1,18,8)
  Demux1 : Demux  Outputs=3
  Demux2 : Demux  Outputs=3
  Product : Product
  Product1 : Product
  Product2 : Product
  Switch : Switch  Threshold=0.5
  Switch1 : Switch  Threshold=0.5
  Out1 : Outport
  wires:
  In1/1 -> Demux1/1
  In2/1 -> Demux2/1
  Y_disable/1 -> Switch/2
  SAD_SSE/1 -> Switch1/2
  Abs/1 -> Add5/1
  Abs1/1 -> Add5/2
  Abs2/1 -> Add6/2
  Add/1 -> Switch/3
  Add1/1 -> Product1/2, Product1/1, Abs1/1
  Add2/1 -> Product2/2, Product2/1, Abs2/1
  Add3/1 -> Add4/1
  Add4/1 -> Switch1/1
  Add5/1 -> Add6/1
  Add6/1 -> Switch1/3
  Constant/1 -> Switch/1
  Demux1/1 -> Add/1
  Demux1/2 -> Add1/1
  Demux1/3 -> Add2/1
  Demux2/1 -> Add/2
  Demux2/2 -> Add1/2
  Demux2/3 -> Add2/2
  Product/1 -> Add3/1
  Product1/1 -> Add3/2
  Product2/1 -> Add4/2
  Switch/1 -> Product/2, Product/1, Abs/1
  Switch1/1 -> Out1/1

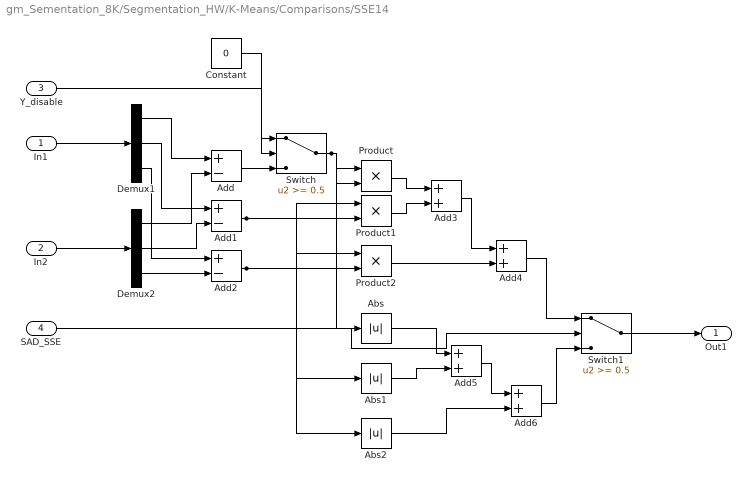
== system gm_Sementation_8K/Segmentation_HW/K-Means/Comparisons/SSE14 ==
  In1 : Inport  OutDataTypeStr=fixdt(1, 18, 8)  PortDimensions=[1 3]  SampleTime=0.001
  In2 : Inport  Port=2  OutDataTypeStr=fixdt(1, 18, 8)  PortDimensions=[1 3]  SampleTime=0.001
  Y_disable : Inport  Port=3  OutDataTypeStr=fixdt(1, 18, 8)  PortDimensions=1
  SAD_SSE : Inport  Port=4  OutDataTypeStr=fixdt(1, 18, 8)  PortDimensions=1
  Abs : Abs
  Abs1 : Abs
  Abs2 : Abs
  Add : Sum  Inputs=+-  OutDataTypeStr=Inherit: Inherit via back propagation
  Add1 : Sum  Inputs=+-  OutDataTypeStr=Inherit: Inherit via back propagation
  Add2 : Sum  Inputs=+-  OutDataTypeStr=Inherit: Inherit via back propagation
  Add{3..6} (4 alike) : Sum
  Constant : Constant  Value=0  OutDataTypeStr=fixdt(1,18,8)
  Demux1 : Demux  Outputs=3
  Demux2 : Demux  Outputs=3
  Product : Product
  Product1 : Product
  Product2 : Product
  Switch : Switch  Threshold=0.5
  Switch1 : Switch  Threshold=0.5
  Out1 : Outport
  wires:
  In1/1 -> Demux1/1
  In2/1 -> Demux2/1
  Y_disable/1 -> Switch/2
  SAD_SSE/1 -> Switch1/2
  Abs/1 -> Add5/1
  Abs1/1 -> Add5/2
  Abs2/1 -> Add6/2
  Add/1 -> Switch/3
  Add1/1 -> Product1/2, Product1/1, Abs1/1
  Add2/1 -> Product2/2, Product2/1, Abs2/1
  Add3/1 -> Add4/1
  Add4/1 -> Switch1/1
  Add5/1 -> Add6/1
  Add6/1 -> Switch1/3
  Constant/1 -> Switch/1
  Demux1/1 -> Add/1
  Demux1/2 -> Add1/1
  Demux1/3 -> Add2/1
  Demux2/1 -> Add/2
  Demux2/2 -> Add1/2
  Demux2/3 -> Add2/2
  Product/1 -> Add3/1
  Product1/1 -> Add3/2
  Product2/1 -> Add4/2
  Switch/1 -> Product/2, Product/1, Abs/1
  Switch1/1 -> Out1/1

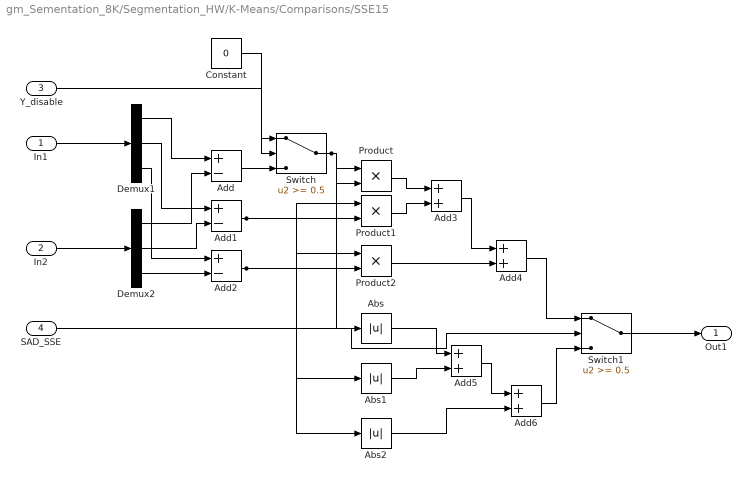
== system gm_Sementation_8K/Segmentation_HW/K-Means/Comparisons/SSE15 ==
  In1 : Inport  OutDataTypeStr=fixdt(1, 18, 8)  PortDimensions=[1 3]  SampleTime=0.001
  In2 : Inport  Port=2  OutDataTypeStr=fixdt(1, 18, 8)  PortDimensions=[1 3]  SampleTime=0.001
  Y_disable : Inport  Port=3  OutDataTypeStr=fixdt(1, 18, 8)  PortDimensions=1
  SAD_SSE : Inport  Port=4  OutDataTypeStr=fixdt(1, 18, 8)  PortDimensions=1
  Abs : Abs
  Abs1 : Abs
  Abs2 : Abs
  Add : Sum  Inputs=+-  OutDataTypeStr=Inherit: Inherit via back propagation
  Add1 : Sum  Inputs=+-  OutDataTypeStr=Inherit: Inherit via back propagation
  Add2 : Sum  Inputs=+-  OutDataTypeStr=Inherit: Inherit via back propagation
  Add{3..6} (4 alike) : Sum
  Constant : Constant  Value=0  OutDataTypeStr=fixdt(1,18,8)
  Demux1 : Demux  Outputs=3
  Demux2 : Demux  Outputs=3
  Product : Product
  Product1 : Product
  Product2 : Product
  Switch : Switch  Threshold=0.5
  Switch1 : Switch  Threshold=0.5
  Out1 : Outport
  wires:
  In1/1 -> Demux1/1
  In2/1 -> Demux2/1
  Y_disable/1 -> Switch/2
  SAD_SSE/1 -> Switch1/2
  Abs/1 -> Add5/1
  Abs1/1 -> Add5/2
  Abs2/1 -> Add6/2
  Add/1 -> Switch/3
  Add1/1 -> Product1/2, Product1/1, Abs1/1
  Add2/1 -> Product2/2, Product2/1, Abs2/1
  Add3/1 -> Add4/1
  Add4/1 -> Switch1/1
  Add5/1 -> Add6/1
  Add6/1 -> Switch1/3
  Constant/1 -> Switch/1
  Demux1/1 -> Add/1
  Demux1/2 -> Add1/1
  Demux1/3 -> Add2/1
  Demux2/1 -> Add/2
  Demux2/2 -> Add1/2
  Demux2/3 -> Add2/2
  Product/1 -> Add3/1
  Product1/1 -> Add3/2
  Product2/1 -> Add4/2
  Switch/1 -> Product/2, Product/1, Abs/1
  Switch1/1 -> Out1/1

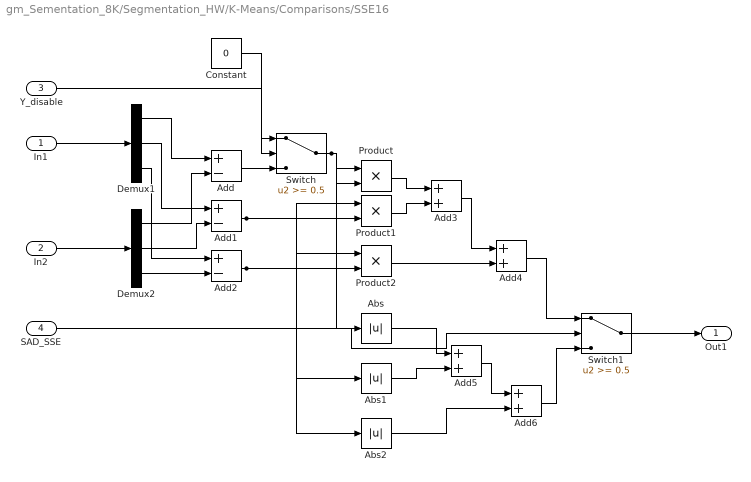
== system gm_Sementation_8K/Segmentation_HW/K-Means/Comparisons/SSE16 ==
  In1 : Inport  OutDataTypeStr=fixdt(1, 18, 8)  PortDimensions=[1 3]  SampleTime=0.001
  In2 : Inport  Port=2  OutDataTypeStr=fixdt(1, 18, 8)  PortDimensions=[1 3]  SampleTime=0.001
  Y_disable : Inport  Port=3  OutDataTypeStr=fixdt(1, 18, 8)  PortDimensions=1
  SAD_SSE : Inport  Port=4  OutDataTypeStr=fixdt(1, 18, 8)  PortDimensions=1
  Abs : Abs
  Abs1 : Abs
  Abs2 : Abs
  Add : Sum  Inputs=+-  OutDataTypeStr=Inherit: Inherit via back propagation
  Add1 : Sum  Inputs=+-  OutDataTypeStr=Inherit: Inherit via back propagation
  Add2 : Sum  Inputs=+-  OutDataTypeStr=Inherit: Inherit via back propagation
  Add{3..6} (4 alike) : Sum
  Constant : Constant  Value=0  OutDataTypeStr=fixdt(1,18,8)
  Demux1 : Demux  Outputs=3
  Demux2 : Demux  Outputs=3
  Product : Product
  Product1 : Product
  Product2 : Product
  Switch : Switch  Threshold=0.5
  Switch1 : Switch  Threshold=0.5
  Out1 : Outport
  wires:
  In1/1 -> Demux1/1
  In2/1 -> Demux2/1
  Y_disable/1 -> Switch/2
  SAD_SSE/1 -> Switch1/2
  Abs/1 -> Add5/1
  Abs1/1 -> Add5/2
  Abs2/1 -> Add6/2
  Add/1 -> Switch/3
  Add1/1 -> Product1/2, Product1/1, Abs1/1
  Add2/1 -> Product2/2, Product2/1, Abs2/1
  Add3/1 -> Add4/1
  Add4/1 -> Switch1/1
  Add5/1 -> Add6/1
  Add6/1 -> Switch1/3
  Constant/1 -> Switch/1
  Demux1/1 -> Add/1
  Demux1/2 -> Add1/1
  Demux1/3 -> Add2/1
  Demux2/1 -> Add/2
  Demux2/2 -> Add1/2
  Demux2/3 -> Add2/2
  Product/1 -> Add3/1
  Product1/1 -> Add3/2
  Product2/1 -> Add4/2
  Switch/1 -> Product/2, Product/1, Abs/1
  Switch1/1 -> Out1/1

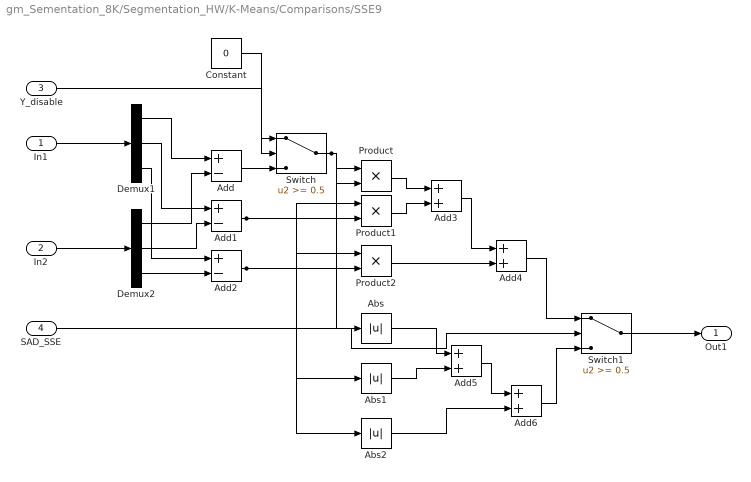
== system gm_Sementation_8K/Segmentation_HW/K-Means/Comparisons/SSE9 ==
  In1 : Inport  OutDataTypeStr=fixdt(1, 18, 8)  PortDimensions=[1 3]  SampleTime=0.001
  In2 : Inport  Port=2  OutDataTypeStr=fixdt(1, 18, 8)  PortDimensions=[1 3]  SampleTime=0.001
  Y_disable : Inport  Port=3  OutDataTypeStr=fixdt(1, 18, 8)  PortDimensions=1
  SAD_SSE : Inport  Port=4  OutDataTypeStr=fixdt(1, 18, 8)  PortDimensions=1
  Abs : Abs
  Abs1 : Abs
  Abs2 : Abs
  Add : Sum  Inputs=+-  OutDataTypeStr=Inherit: Inherit via back propagation
  Add1 : Sum  Inputs=+-  OutDataTypeStr=Inherit: Inherit via back propagation
  Add2 : Sum  Inputs=+-  OutDataTypeStr=Inherit: Inherit via back propagation
  Add{3..6} (4 alike) : Sum
  Constant : Constant  Value=0  OutDataTypeStr=fixdt(1,18,8)
  Demux1 : Demux  Outputs=3
  Demux2 : Demux  Outputs=3
  Product : Product
  Product1 : Product
  Product2 : Product
  Switch : Switch  Threshold=0.5
  Switch1 : Switch  Threshold=0.5
  Out1 : Outport
  wires:
  In1/1 -> Demux1/1
  In2/1 -> Demux2/1
  Y_disable/1 -> Switch/2
  SAD_SSE/1 -> Switch1/2
  Abs/1 -> Add5/1
  Abs1/1 -> Add5/2
  Abs2/1 -> Add6/2
  Add/1 -> Switch/3
  Add1/1 -> Product1/2, Product1/1, Abs1/1
  Add2/1 -> Product2/2, Product2/1, Abs2/1
  Add3/1 -> Add4/1
  Add4/1 -> Switch1/1
  Add5/1 -> Add6/1
  Add6/1 -> Switch1/3
  Constant/1 -> Switch/1
  Demux1/1 -> Add/1
  Demux1/2 -> Add1/1
  Demux1/3 -> Add2/1
  Demux2/1 -> Add/2
  Demux2/2 -> Add1/2
  Demux2/3 -> Add2/2
  Product/1 -> Add3/1
  Product1/1 -> Add3/2
  Product2/1 -> Add4/2
  Switch/1 -> Product/2, Product/1, Abs/1
  Switch1/1 -> Out1/1

== matlab function gm_Sementation_8K/Segmentation_HW/K-Means/Clustering/MATLAB Function/MATLAB Function ==
  data: vstart input; fr_num input; addr input; rgb input; RGB0 output fixdt(1,18,8) size=[1,3]; rgb0 input; rgb1 input; RGB1 output fixdt(1,18,8) size=[1,3]; rgb2 input; rgb3 input; RGB2 output fixdt(1,18,8) size=[1,3]; RGB3 output fixdt(1,18,8) size=[1,3]; rgb4 input; rgb5 input; rgb6 input; rgb7 input; RGB4 output fixdt(1,18,8) size=[1,3]; RGB5 output fixdt(1,18,8) size=[1,3]; RGB6 output fixdt(1,18,8) size=[1,3]; RGB7 output fixdt(1,18,8) size=[1,3]
function [RGB0,RGB1,RGB2,RGB3,RGB4,RGB5,RGB6,RGB7] = fcn(vstart,fr_num,addr,rgb,rgb0,rgb1,rgb2,rgb3,rgb4,rgb5,rgb6,rgb7)

alpha = fi(0.999);
rgb_alpha = (rgb)*fi(fi(1)-alpha);
rgb00 = fi(rgb0,1,18,8);
rgb11 = fi(rgb1,1,18,8);
rgb22 = fi(rgb2,1,18,8);
rgb33 = fi(rgb3,1,18,8);
rgb44 = fi(rgb4,1,18,8);
rgb55 = fi(rgb5,1,18,8);
rgb66 = fi(rgb6,1,18,8);
rgb77 = fi(rgb7,1,18,8);

if(vstart&(fr_num==0))
    RGB00 = fi([127,127,127],1,18,8);
    RGB11 = fi([127,127,127],1,18,8);
    RGB22 = fi([100,127,127],1,18,8);
    RGB33 = fi([127,127,127],1,18,8);
    RGB44 = fi([127,127,127],1,18,8);
    RGB55 = fi([127,127,127],1,18,8);
    RGB66 = fi([127,127,127],1,18,8);
    RGB77 = fi([127,127,127],1,18,8);
else
    if(addr==0)
        RGB00 = fi(rgb00*alpha + rgb_alpha,1,18,8);
        RGB11 = rgb11;
        RGB22 = rgb22;
        RGB33 = rgb33;
        RGB44 = rgb44;
        RGB55 = rgb55;
        RGB66 = rgb66;
        RGB77 = rgb77;
    elseif(addr==1)
        RGB00 = rgb00;
        RGB11 = fi(rgb11*alpha + rgb_alpha,1,18,8);
        RGB22 = rgb22;
        RGB33 = rgb33;
        RGB44 = rgb44;
        RGB55 = rgb55;
        RGB66 = rgb66;
        RGB77 = rgb77;
    elseif(addr==2)
        RGB00 = rgb00;
        RGB11 = rgb11;
        RGB22 = fi(rgb22*alpha + rgb_alpha,1,18,8);
        RGB33 = rgb33;
        RGB44 = rgb44;
        RGB55 = rgb55;
        RGB66 = rgb66;
        RGB77 = rgb77;
    elseif(addr==3)
        RGB00 = rgb00;
        RGB11 = rgb11;
        RGB22 = rgb22;
        RGB33 = fi(rgb33*alpha + rgb_alpha,1,18,8);
        RGB44 = rgb44;
        RGB55 = rgb55;
        RGB66 = rgb66;
        RGB77 = rgb77;
    elseif(addr==4)
        RGB00 = rgb00;
        RGB11 = rgb11;
        RGB22 = rgb22;
        RGB33 = rgb33;
        RGB44 = fi(rgb44*alpha + rgb_alpha,1,18,8);
        RGB55 = rgb55;
        RGB66 = rgb66;
        RGB77 = rgb77;
    elseif(addr==5)
        RGB00 = rgb00;
        RGB11 = rgb11;
        RGB22 = rgb22;
        RGB33 = rgb33;
        RGB44 = rgb44;
        RGB55 = fi(rgb55*alpha + rgb_alpha,1,18,8);
        RGB66 = rgb66;
        RGB77 = rgb77;
    elseif(addr==6)
        RGB00 = rgb00;
        RGB11 = rgb11;
        RGB22 = rgb22;
        RGB33 = rgb33;
        RGB44 = rgb44;
        RGB55 = rgb55;
        RGB66 = fi(rgb66*alpha + rgb_alpha,1,18,8);
        RGB77 = rgb77;
    else
        RGB00 = rgb00;
        RGB11 = rgb11;
        RGB22 = rgb22;
        RGB33 = rgb33;
        RGB44 = rgb44;
        RGB55 = rgb55;
        RGB66 = rgb66;
        RGB77 = fi(rgb77*alpha + rgb_alpha,1,18,8);
    end
end

RGB0 = fi(RGB00,1,18,8);
RGB1 = fi(RGB11,1,18,8);
RGB2 = fi(RGB22,1,18,8);
RGB3 = fi(RGB33,1,18,8);
RGB4 = fi(RGB44,1,18,8);
RGB5 = fi(RGB55,1,18,8);
RGB6 = fi(RGB66,1,18,8);
RGB7 = fi(RGB77,1,18,8);

== matlab function gm_Sementation_8K/Segmentation_SW ==
  data: img_in input; img_out output
function img_out = fcn(img_in)
wl = 18;
fr = 8;
k_cnt = 8;
persistent k;
k = fi(ones(k_cnt,3)*127,1,wl,fr);
k_out = fi([255,0,0;0,255,0;0,0,255;255,255,0;0,255,255;255,0,255;0,0,0;255,255,255],1,wl,fr);
alpha = fi(0.999);
s = size(img_in);
img_in = rgb2ycbcr(img_in);
% img_out = img_in;

for i=1:s(1)
    for j=1:s(2)
        in = img_in(i,j,:);
        in = [in(1),in(2),in(3)];
        p = repmat(in,k_cnt,1);
        p = fi(p,1,wl,fr);
        %Find closest matching cluster centroid using SAD
        scores = abs(p-k);
        scores = sum(scores(:,2:3),2);  %Skip Y in the first column
        [Y,adr] = min(scores);
        img_in(i,j,:) = k(adr,:);
        %Update matched centroid
        k(adr,:) = k(adr,:)*alpha + (1-alpha)*in;
    end
%     i*100/s(1)
end
img_out = uint8(img_in);
img_out = ycbcr2rgb(img_out);
